simulink model "c9mimp3"  (R2022a)
settings: Solver=ode45  StartTime=0.0  StopTime=10.0  RelTol=1e-10
PreLoadFcn:
  | ww=[1e-6 1e6]; N=35;
libraries: cstblocks x1
settings Model: Creator=xuedi  LastModifiedBy=xuedi
settings DataIOCC: SaveFormat=Array  ReturnWorkspaceOutputs=off

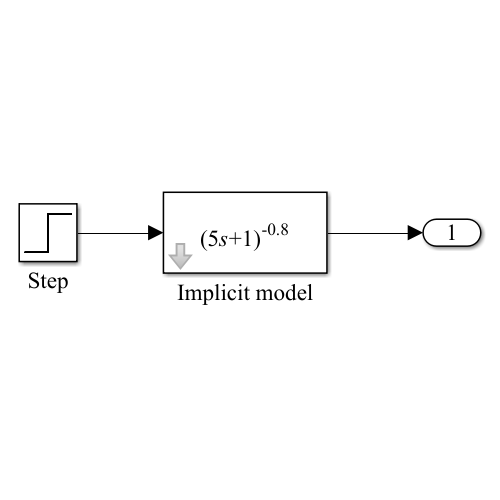
[thumbnail: Simulink's stored preview of the top-level diagram]
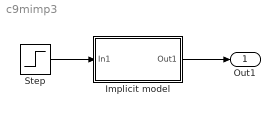
== system c9mimp3 ==
  Implicit model : Subsystem  mask{tau=5, nu=0.8, ww=ww, N=N, keyCD=Continous}
      mask prompts: tau "Time constant tau"; nu "power nu"; ww "Frequency range [wb,wh]"; N "Filter order"; keyCD "Filter type"
      mask init:
      | str=['(' num2str(tau) '{\its}+1)^{' num2str(-nu) '}'];
      |    if keyCD==1, G=tf(1,1);
      |    else, T=ww(1); G=irid_folpf(tau,nu,T,N); end
      mask TypeOptions keyCD: Continous | Discrete Filter
      mask Display: disp(str,'texmode','on')
  Step : Step  Time=0  SampleTime=0
  Out1 : Outport
  wires:
  Step/1 -> Implicit model/1(In1)
  Implicit model/1(Out1) -> Out1/1

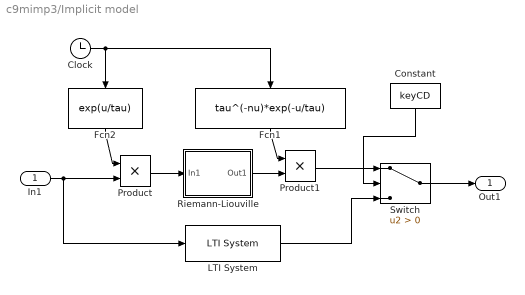
== system c9mimp3/Implicit model ==
  In1 : Inport
  Clock : Clock
  Constant : Constant  Value=keyCD
  Fcn1 : Fcn  Expr=tau^(-nu)*exp(-u/tau)
  Fcn2 : Fcn  Expr=exp(u/tau)
  LTI System : cstblocks/LTI System  sys=G  IC=[]
  Product : Product
  Product1 : Product
  "Riemann-Liouville " : Subsystem  mask{gam=-nu, ww=ww, n=N, kF1=on, kF=Oustaloup filter}
      mask prompts: gam "Derivative order gamma"; ww "Frequency range [wb,wh]"; n "Apprixmation order"; kF1 "Is a low-pass filter required?"; kF "Filter type"
      mask init:
      | wb=ww(1); wh=ww(2); 
      | if kF==1, G=ousta_fod(gam,n,wb,wh);
      | else, G=new_fod(gam,n,wb,wh); end
      | G=tf(G); num=G.num{1}; den=G.den{1}; T=1/wh; 
      | if isnumeric(gam), str=['{\its}^{' num2str(gam) '}']; 
      | else, str='{\its}^{gam}'; end
      | if kF1==1, G=G*tf(1,[T 1]); end
      mask TypeOptions kF: Oustaloup filter | Modified Oustaloup filter | Matsuda-Fujii filter
      mask Display: disp(str,'texmode','on')
  Switch : Switch  Criteria=u2 > Threshold  SaturateOnIntegerOverflow=off  InputSameDT=off
  Out1 : Outport
  wires:
  Clock/1 -> Fcn1/1, Fcn2/1
  Fcn1/1 -> Product1/1
  "Riemann-Liouville "/1(Out1) -> Product1/2
  Product/1 -> "Riemann-Liouville "/1(In1)
  Fcn2/1 -> Product/1
  Product1/1 -> Switch/1
  Switch/1 -> Out1/1
  Constant/1 -> Switch/2
  In1/1 -> LTI System/1, Product/2
  LTI System/1 -> Switch/3

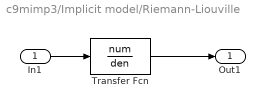
== system c9mimp3/Implicit model/Riemann-Liouville  ==
  In1 : Inport
  Transfer Fcn : TransferFcn  Numerator=num  Denominator=den
  Out1 : Outport
  wires:
  In1/1 -> Transfer Fcn/1
  Transfer Fcn/1 -> Out1/1
